simulink model "sample02_current_mode_angle_p_I2C0_0x64_and_0x65"  (R2025a)
settings: Solver=ode1  StartTime=0.0  StopTime=inf  FixedStep=0.005  RelTol=1e-3  EnableMultiTasking=on
libraries: roller485lib x6
settings Model: SILPILModeSetting=veronly  ExtModeTrigDuration=2  Creator=kawata  LastModifiedBy=kawata
settings SolverCC: AutoInsertRateTranBlk=on
settings DataIOCC: ReturnWorkspaceOutputs=off
settings OptimizationCC: EnhancedBackFolding=on  PassReuseOutputArgsAs=Individual arguments  ZeroExternalMemoryAtStartup=off  ZeroInternalMemoryAtStartup=off  MaxStackSize=64  OptimizeBlockOrder=speed  DifferentSizesBufferReuse=on  OptimizationCustomize=off  EfficientTunableParamExpr=on
settings DebuggingCC: ParameterTunabilityLossMsg=error
settings HardwareCC: ProdBitPerPointer=32.0  ProdBitPerSizeT=32.0  ProdBitPerPtrDiffT=32.0  ProdLargestAtomicInteger=Long  ProdLargestAtomicFloat=Double  ProdWordSize=32.0  ProdHWDeviceType=ARM Compatible->ARM Cortex  UseEmbeddedCoderFeatures=off  UseSimulinkCoderFeatures=off
settings SFSimCC: MATLABDynamicMemAlloc=off
settings RTWCC: SystemTargetFile=ert.tlc  HardwareBoard=Raspberry Pi Pico (Arduino Compatible)  TLCOptions="-aInlineSetEventsForThisBaseRateFcn=TLC_FALSE -aSuppressMultiTaskScheduler=TLC_FALSE   -aRateBasedStepFcn=1"  TemplateMakefile=ert_default_tmf  Toolchain=Arduino ARM RP2040  BuildConfiguration=Faster Runs  Description=Embedded Coder
settings CodeAppCC: ForceParamTrailComments=on  IgnoreCustomStorageClasses=off  OperatorAnnotations=on  SimulinkDataObjDesc=on  SFDataObjDesc=on  InsertBlockDesc=on
settings ERTTargetCC: ExtModeTransport=3.0  ExtModeAutomaticAllocSize=off  ExtModeStaticAllocSize=65536.0  InlinedParameterPlacement=Hierarchical  SupportContinuousTime=on  SupportNonInlinedSFcns=on  SupportVariableSizeSignals=on

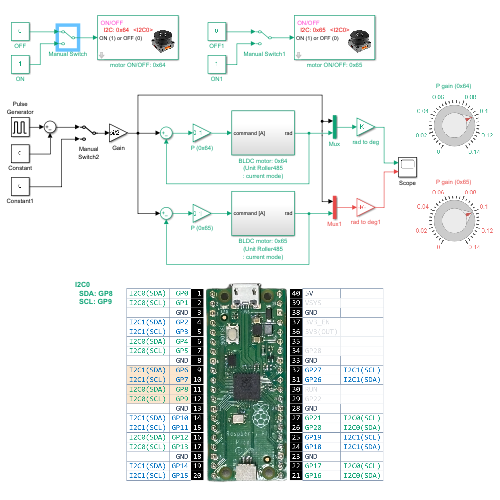
[thumbnail: Simulink's stored preview of the top-level diagram]
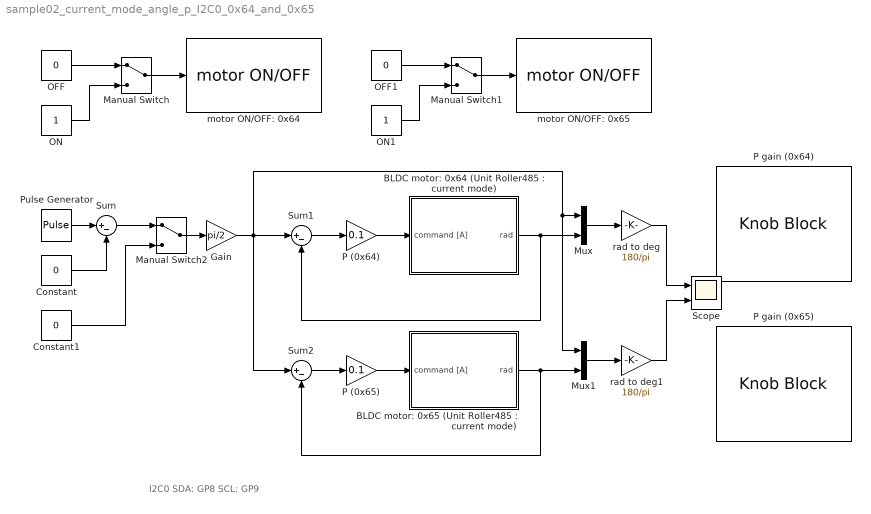
== system sample02_current_mode_angle_p_I2C0_0x64_and_0x65 ==
  note: I2C0
      | SDA: GP8
      | SCL: GP9
  "BLDC motor: 0x64 (Unit Roller485 : current mode)" : Subsystem
  "BLDC motor: 0x65 (Unit Roller485 : current mode)" : Subsystem
  Constant : Constant  Value=0
  Constant1 : Constant  Value=0
  Gain : Gain  Gain=pi/2
  Manual Switch2 : ManualSwitch
  Manual Switch : ManualSwitch
  Manual Switch1 : ManualSwitch
  Mux : Mux  Inputs=2
  Mux1 : Mux  Inputs=2
  OFF : Constant  Value=0
  OFF1 : Constant  Value=0
  ON : Constant
  ON1 : Constant
  P (0x64) : Gain  Gain=0.1
  P (0x65) : Gain  Gain=0.1
  P gain (0x64) : KnobBlock  LabelPosition=Hide  ScaleMax=0.14  TickInterval=0.02
  P gain (0x65) : KnobBlock  LabelPosition=Hide  ScaleMax=0.14  TickInterval=0.02
  Pulse Generator : DiscretePulseGenerator  PulseType=Time based  Period=4  PulseWidth=50  PhaseDelay=1
  Scope : Scope  NumInputPorts=2
      settings: TimeSpan=4  ActiveDisplayYMinimum=-45  ActiveDisplayYMaximum=135
  Sum : Sum  Inputs=|+-
  Sum1 : Sum  Inputs=|+-
  Sum2 : Sum  Inputs=|+-
  motor ON/OFF: 0x64 : roller485lib/motor ON//OFF  I2CAddress=0x64  I2CModule=0
      settings: SourceProductName=Roller485 Library
  motor ON/OFF: 0x65 : roller485lib/motor ON//OFF  I2CAddress=0x65  I2CModule=0
      settings: SourceProductName=Roller485 Library
  rad to deg : Gain  Gain=180/pi
  rad to deg1 : Gain  Gain=180/pi
  wires:
  Manual Switch/1 -> motor ON/OFF: 0x64/1
  OFF/1 -> Manual Switch/1
  ON/1 -> Manual Switch/2
  Constant/1 -> Sum/2
  Pulse Generator/1 -> Sum/1
  Mux/1 -> rad to deg/1
  P (0x64)/1 -> "BLDC motor: 0x64 (Unit Roller485 : current mode)"/1(command [A])
  Gain/1 -> Sum2/1, Mux1/1, Mux/1, Sum1/1
  "BLDC motor: 0x64 (Unit Roller485 : current mode)"/1(rad) -> Sum1/2, Mux/2
  Manual Switch2/1 -> Gain/1
  Sum/1 -> Manual Switch2/1
  Constant1/1 -> Manual Switch2/2
  Sum1/1 -> P (0x64)/1
  Sum2/1 -> P (0x65)/1
  P (0x65)/1 -> "BLDC motor: 0x65 (Unit Roller485 : current mode)"/1(command [A])
  ON1/1 -> Manual Switch1/2
  OFF1/1 -> Manual Switch1/1
  Manual Switch1/1 -> motor ON/OFF: 0x65/1
  Mux1/1 -> rad to deg1/1
  "BLDC motor: 0x65 (Unit Roller485 : current mode)"/1(rad) -> Mux1/2, Sum2/2
  rad to deg/1 -> Scope/1
  rad to deg1/1 -> Scope/2

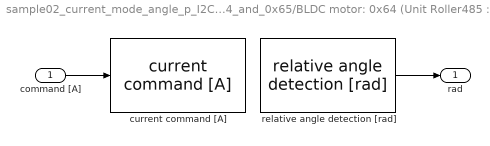
== system sample02_current_mode_angle_p_I2C0_0x64_and_0x65/BLDC motor: 0x64 (Unit Roller485 : current mode) ==
  command [A] : Inport
  current command [A] : roller485lib/I2C Write/current command [A]  I2CAddress=0x64  I2CModule=0  set_time=0
      settings: SourceProductName=Roller485 Library
  relative angle detection [rad] : roller485lib/I2C Read/relative angle detection [rad]  I2CAddress=0x64  I2CModule=0  sample_time=-1  set_time=0
      settings: SourceProductName=Roller485 Library
  rad : Outport
  wires:
  command [A]/1 -> current command [A]/1
  relative angle detection [rad]/1 -> rad/1

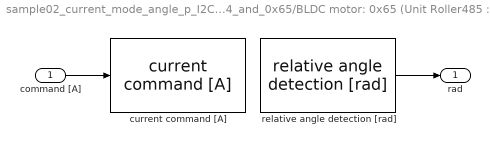
== system sample02_current_mode_angle_p_I2C0_0x64_and_0x65/BLDC motor: 0x65 (Unit Roller485 : current mode) ==
  command [A] : Inport
  current command [A] : roller485lib/I2C Write/current command [A]  I2CAddress=0x65  I2CModule=0  set_time=0
      settings: SourceProductName=Roller485 Library
  relative angle detection [rad] : roller485lib/I2C Read/relative angle detection [rad]  I2CAddress=0x65  I2CModule=0  sample_time=-1  set_time=0
      settings: SourceProductName=Roller485 Library
  rad : Outport
  wires:
  relative angle detection [rad]/1 -> rad/1
  command [A]/1 -> current command [A]/1
